simulink model "diabetes_2sim"  (R2023a)
settings: Solver=ode45  StartTime=0.0  StopTime=24  RelTol=1e-3  EnableMultiTasking=on
StopFcn:
  | plot_results
libraries: simulink x2, realtime_pacer_lib x1
settings Model: Creator=tsladeche  LastModifiedBy=jazbo
settings SolverCC: AlgebraicLoopSolver=TrustRegion
settings DataIOCC: LimitDataPoints=on  SaveFormat=Array  SignalLoggingSaveFormat=ModelDataLogs  ReturnWorkspaceOutputs=off
settings OptimizationCC: ExpressionDepthLimit=2147483647  LifeSpan=inf
settings DebuggingCC: UnderspecifiedInitializationDetection=Classic  MergeDetectMultiDrivingBlocksExec=none  SolverPrmCheckMsg=warning  FcnCallInpInsideContextMsg=warning  UnconnectedInputMsg=warning  UnconnectedOutputMsg=warning  UnconnectedLineMsg=warning  StateNameClashWarn=warning  SFUnexpectedBacktrackingDiag=warning  SFNoUnconditionalDefaultTransitionDiag=warning  SFExecutionAtInitializationDiag=none  ArithmeticOperatorsInVariantConditions=warning
settings HardwareCC: ProdBitPerPointer=32  ProdBitPerSizeT=32  ProdBitPerPtrDiffT=32  ProdLargestAtomicFloat=None  ProdIntDivRoundTo=Undefined  ProdEndianess=Unspecified  ProdWordSize=32  ProdHWDeviceType=32-bit Generic
settings ModelReferenceCC: PropagateSignalLabelsOutOfModel=off
settings SFSimCC: SimUseLocalCustomCode=off  CustomCodeUndefinedFunction=UseInterfaceOnly
settings RTWCC: RTWUseLocalCustomCode=off
settings CodeAppCC: StateflowObjectComments=on
settings GRTTargetCC: TargetLangStandard=C89/C90 (ANSI)  CombineOutputUpdateFcns=off  GRTInterface=on
settings ConfigComp: CovMetricSettings=dw  CovSaveCumulativeToWorkspaceVar=on  CovSaveSingleToWorkspaceVar=on  CovExternalEMLEnable=off

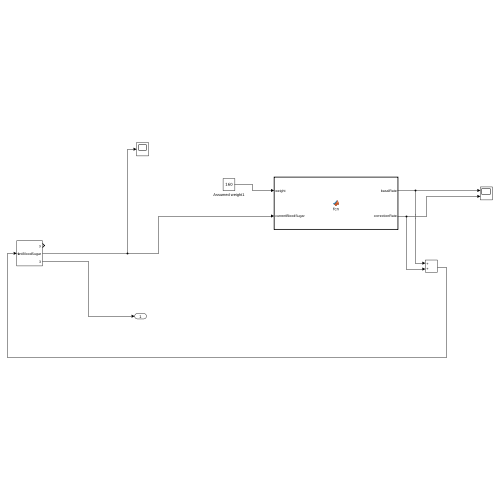
[thumbnail: Simulink's stored preview of the top-level diagram]
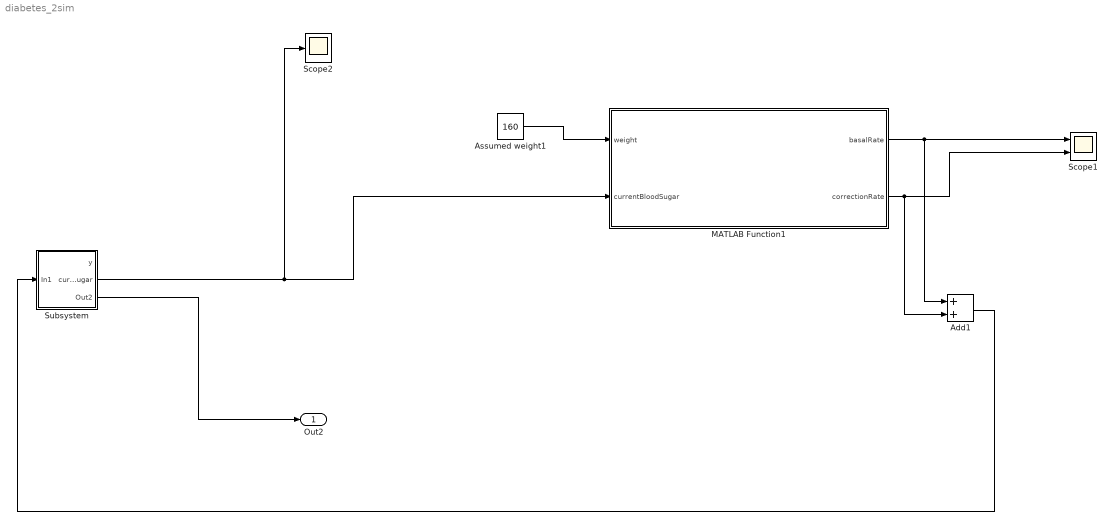
== system diabetes_2sim ==
  Add1 : Sum
  Assumed weight1 : Constant  Value=160
  MATLAB Function1 : MATLAB Function  TreatAsAtomicUnit=on
  Scope1 : Scope  NumInputPorts=2
  Scope2 : Scope
  Subsystem : Subsystem
  Out2 : Outport
  wires:
  Subsystem/3(Out2) -> Out2/1
  MATLAB Function1/1(basalRate) -> Add1/1, Scope1/1
  MATLAB Function1/2(correctionRate) -> Add1/2, Scope1/2
  Subsystem/2(currentBloodSugar) -> MATLAB Function1/2(currentBloodSugar), Scope2/1
  Assumed weight1/1 -> MATLAB Function1/1(weight)
  Add1/1 -> Subsystem/1(In1)

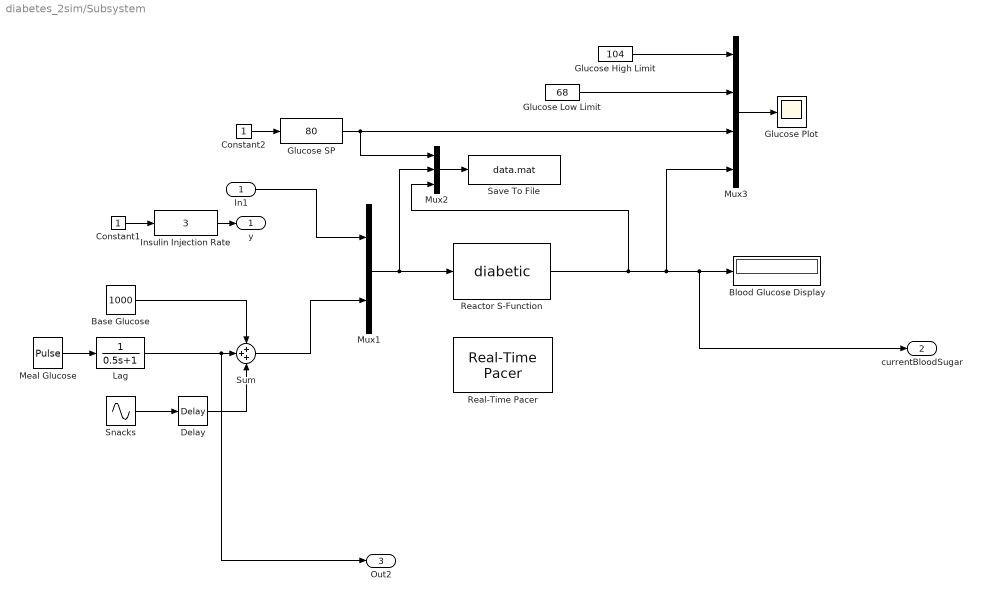
== system diabetes_2sim/Subsystem ==
  In1 : Inport
  Base Glucose : Constant  Value=1000
  Blood Glucose Display : Display
  Constant1 : Constant
  Constant2 : Constant
  Delay : TransportDelay  DelayTime=8
  Glucose High Limit : Constant  Value=104
  Glucose Low Limit : Constant  Value=68
  Glucose Plot : Scope
  Glucose SP : simulink/Math Operations/Slider Gain  gain=80  low=50  high=120
  Insulin Injection Rate : simulink/Math Operations/Slider Gain  gain=3  low=0  high=10
  Lag : TransferFcn  Denominator=[0.5 1]
  Meal Glucose : DiscretePulseGenerator  PulseType=Time based  Amplitude=1000  Period=6  PulseWidth=10  PhaseDelay=7
  Mux1 : Mux  Inputs=2
  Mux2 : Mux  Inputs=3
  Mux3 : Mux
  Reactor S-Function : S-Function  FunctionName=diabetic  SFunctionDeploymentMode=off  EnableBusSupport=off
  Real-Time Pacer : realtime_pacer_lib/Real-Time Pacer  simTimePerRealTime=1
      settings: SourceProductName=Real-Time Pacer
  Save To File : ToFile  Filename=data.mat  MatrixName=diabetic  SampleTime=0.05
  Snacks : Sin  Amplitude=50  SampleTime=0
  Sum : Sum  Inputs=+++
  y : Outport
  currentBloodSugar : Outport  Port=2
  Out2 : Outport  Port=3
  wires:
  Snacks/1 -> Delay/1
  Sum/1 -> Mux1/2
  Reactor S-Function/1 -> Mux3/4, currentBloodSugar/1, Blood Glucose Display/1, Mux2/3
  Meal Glucose/1 -> Lag/1
  Insulin Injection Rate/1 -> y/1
  Constant1/1 -> Insulin Injection Rate/1
  Mux1/1 -> Mux2/2, Reactor S-Function/1
  Constant2/1 -> Glucose SP/1
  Glucose SP/1 -> Mux3/3, Mux2/1
  Base Glucose/1 -> Sum/1
  Delay/1 -> Sum/3
  In1/1 -> Mux1/1
  Glucose Low Limit/1 -> Mux3/2
  Lag/1 -> Out2/1, Sum/2
  Mux3/1 -> Glucose Plot/1
  Mux2/1 -> Save To File/1
  Glucose High Limit/1 -> Mux3/1

== matlab function diabetes_2sim/MATLAB Function1 ==
  data: weight input; basalRate output; currentBloodSugar input; correctionRate output
function [basalRate, correctionRate]= fcn(weight, currentBloodSugar)

    % Constants
    TARGET_BLOOD_SUGAR = 100; % Target blood sugar level in mg/dl
    CORRECTION_FACTOR_CONSTANT = 1800; % Constant for correction factor calculation

    % Total Daily Insulin Dose (TDI)
    totalDailyInsulin = weight / 4;

    % Basal/background Insulin Dose
    basalDose = 0.5 * totalDailyInsulin; % 50% of TDI

    % Basal Insulin Delivery Rate per min
    basalRate = basalDose / 24 / 60; % Delivery rate per minute

    % Correction Factor
    correctionFactor = CORRECTION_FACTOR_CONSTANT / totalDailyInsulin;

    % Correction Dose Calculation
    if currentBloodSugar > 120 % High blood sugar state
        correctionDose = (currentBloodSugar - TARGET_BLOOD_SUGAR) / correctionFactor;
    elseif currentBloodSugar < 80 % Low blood sugar state
        basalRate = 0; % Suspend basal insulin delivery
        correctionDose = 0;
    else
        correctionDose = 0; % Normal blood sugar state
    end
    
    correctionRate = correctionDose % Correction Rate per minute
    
end
